simulink model "PaperMachine"  (Simulink 7.0)
settings: Solver=ode45  StartTime=0.0  StopTime=30.0  RelTol=1e-3
libraries: mpclib x1
settings Model: Creator=rchen  LastModifiedBy=rchen
settings DataIOCC: SignalLoggingName=sigsOut
settings OptimizationCC: InlineInvariantSignals=on
settings DebuggingCC: SaveWithParameterizedLinksMsg=none  CheckExecutionContextPreStartOutputMsg=on  CheckExecutionContextRuntimeOutputMsg=on  SignalResolutionControl=TryResolveAllWithWarning  SolverPrmCheckMsg=none  MultiTaskDSMMsg=warning  MultiTaskCondExecSysMsg=none  StrictBusMsg=None
settings HardwareCC: TargetUnknown=on
settings RTWCC: IncludeERTFirstTime=on
settings GRTTargetCC: TargetFcnLib=ansi_tfl_tmw.mat

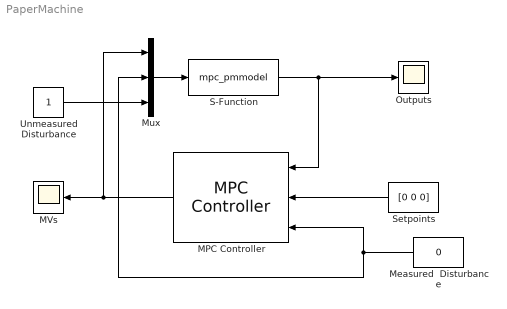
== system PaperMachine ==
  MPC Controller : mpclib/MPC Controller  Orientation=left  SystemSampleTime=-1  mpcobj=MPC1  n_mv=0  x0=[]  ref_from_ws=off  ref_signal_name=[]  ref_preview=on  md_from_ws=off  md_signal_name=[]  md_preview=on  from_project=off  md_inport=on  mv_inport=off  lims_inport=off  project_file=MPCtask.mat
  MVs : Scope
  Measured  Disturbance : Constant  Orientation=left  Value=0  OutDataType=sfix(16)  OutScaling=2^0
  Mux : Mux  Inputs=3
  Outputs : Scope
  S-Function : S-Function  FunctionName=mpc_pmmodel  EnableBusSupport=off
  Setpoints : Constant  Orientation=left  Value=[0 0 0]  OutDataType=sfix(16)  OutScaling=2^0
  Unmeasured Disturbance : Constant  OutDataType=sfix(16)  OutScaling=2^0
  wires:
  S-Function/1 -> Outputs/1, MPC Controller/1
  Setpoints/1 -> MPC Controller/2
  Measured  Disturbance/1 -> Mux/2, MPC Controller/3
  Mux/1 -> S-Function/1
  MPC Controller/1 -> Mux/1, MVs/1
  Unmeasured Disturbance/1 -> Mux/3
